simulink model "run_targeting"  (R2020a)
settings: Solver=ode23  StartTime=0.0  StopTime=7  MaxStep=0.01  RelTol=1e-6  EnableMultiTasking=on
InitFcn:
  | addpath('display/')
  | addpath('parameters/')
  | addpath('quadrotor_model')
  | addpath('tools/')
  | addpath('libs/RealTima_Pacer')
  | aerosonde_parameters
  | simulation_parameters
undefined symbols (not defined in the file or in its folder): drawQuadrotor, filter_freq, plotmavstatevariables, SAMPLE_TIME
libraries: simulink x23, realtime_pacer_lib x1
settings Model: Creator=beard  LastModifiedBy=andrey
settings DataIOCC: LimitDataPoints=on  SaveFormat=Array  SignalLoggingSaveFormat=ModelDataLogs  ReturnWorkspaceOutputs=off
settings OptimizationCC: ExpressionDepthLimit=2147483647  InitFltsAndDblsToZero=on  LifeSpan=inf
settings DebuggingCC: UnderspecifiedInitializationDetection=Classic  MergeDetectMultiDrivingBlocksExec=none  SolverPrmCheckMsg=warning  FcnCallInpInsideContextMsg=warning  AllowSymbolicDim=off  StateNameClashWarn=warning  SFUnexpectedBacktrackingDiag=warning  SFNoUnconditionalDefaultTransitionDiag=warning  SFExecutionAtInitializationDiag=none  ArithmeticOperatorsInVariantConditions=warning
settings HardwareCC: ProdBitPerPointer=32  ProdBitPerSizeT=32  ProdBitPerPtrDiffT=32  ProdLargestAtomicFloat=None  ProdIntDivRoundTo=Undefined  ProdEndianess=Unspecified  ProdWordSize=32  ProdHWDeviceType=32-bit Generic
settings ModelReferenceCC: PropagateSignalLabelsOutOfModel=off
settings SFSimCC: SimUseLocalCustomCode=off  CustomCodeUndefinedFunction=UseInterfaceOnly
settings RTWCC: RTWUseLocalCustomCode=off
settings CodeAppCC: StateflowObjectComments=on
settings GRTTargetCC: TargetLangStandard=C89/C90 (ANSI)  CombineOutputUpdateFcns=off  GRTInterface=on
settings ConfigComp: CovMetricSettings=dw  CovSaveCumulativeToWorkspaceVar=on  CovSaveSingleToWorkspaceVar=on  CovExternalEMLEnable=off  CovSFcnEnable=off

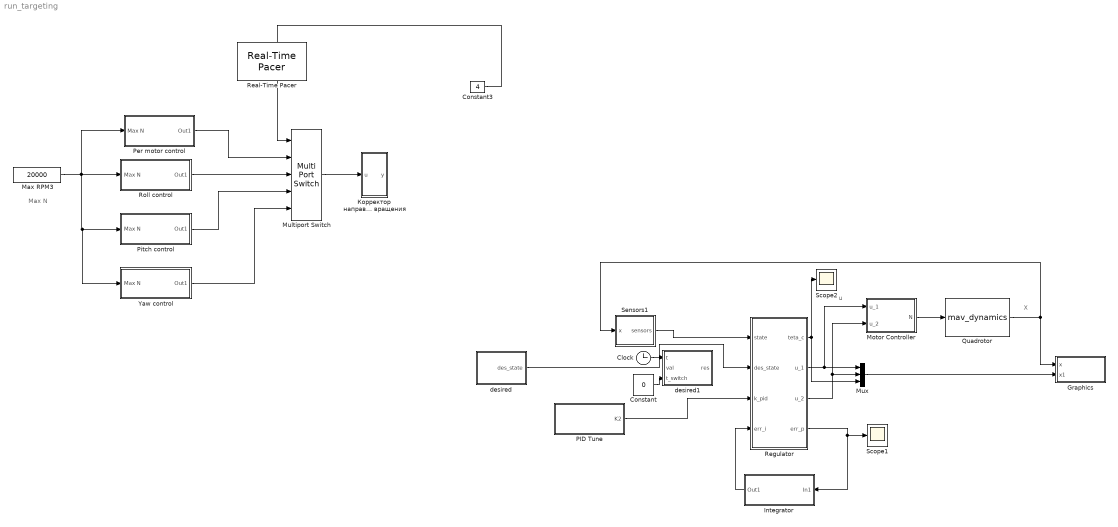
== system run_targeting ==
  note: X
  note: Max N
  note: u
  Clock : Clock
  Constant : Constant  Value=0
  Constant3 : Constant  Value=4
  Graphics : Subsystem
      mask Display: image(imread('../chap2/tv.jpg'))
  Integrator : Subsystem
  Max RPM3 : Constant  Value=20000  SampleTime=SAMPLE_TIME
  Motor Controller : MATLAB Function  TreatAsAtomicUnit=on
  Multiport Switch : MultiPortSwitch  Inputs=4
  Mux : Mux  Inputs=3
  PID Tune : Subsystem
  Per motor control : Subsystem
  Pitch control : Subsystem
  Quadrotor : S-Function  FunctionName=mav_dynamics  Parameters=MAV  SFunctionDeploymentMode=off  EnableBusSupport=off
  Real-Time Pacer : realtime_pacer_lib/Real-Time Pacer  simTimePerRealTime=1
  Regulator : MATLAB Function  TreatAsAtomicUnit=on
  Roll control : Subsystem
  Scope1 : Scope
  Scope2 : Scope
  Sensors1 : Subsystem
  Yaw control : Subsystem
  desired : MATLAB Function  TreatAsAtomicUnit=on
  desired1 : MATLAB Function  TreatAsAtomicUnit=on
  Корректор направлений вращения : MATLAB Function  TreatAsAtomicUnit=on
  wires:
  Quadrotor/1 -> Sensors1/1("x "), Graphics/1(x)
  Max RPM3/1 -> Roll control/1(Max N), Yaw control/1(Max N), Pitch control/1(Max N), Per motor control/1(Max N)
  Constant3/1 -> Multiport Switch/1
  Multiport Switch/1 -> Корректор направлений вращения/1(u)
  Per motor control/1(Out1) -> Multiport Switch/2
  Roll control/1(Out1) -> Multiport Switch/3
  Pitch control/1(Out1) -> Multiport Switch/4
  Yaw control/1(Out1) -> Multiport Switch/5
  Regulator/3(u_2) -> Motor Controller/2(u_2), Mux/2
  Regulator/2(u_1) -> Motor Controller/1(u_1), Mux/1
  Sensors1/1(sensors) -> Regulator/1(state)
  Motor Controller/1(N) -> Quadrotor/1
  Regulator/4(err_p) -> Integrator/1(In1), Scope1/1
  Regulator/1(teta_c) -> Mux/3, Scope2/1
  Integrator/1(Out1) -> Regulator/4(err_i)
  Mux/1 -> Graphics/2(x1)
  Clock/1 -> desired1/1(t)
  Constant/1 -> desired1/3(t_switch)
  PID Tune/1(K2) -> Regulator/3(k_pid)
  desired/1(des_state) -> Regulator/2(des_state)

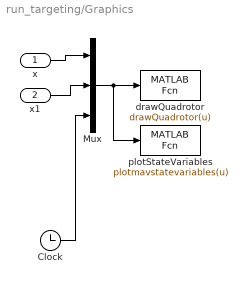
== system run_targeting/Graphics ==
  x : Inport
  x1 : Inport  Port=2
  Clock : Clock
  Mux : Mux  Inputs=3
  drawQuadrotor : MATLABFcn  MATLABFcn=drawQuadrotor(u)  OutputDimensions=0  SampleTime=0.1
  plotStateVariables : MATLABFcn  MATLABFcn=plotmavstatevariables(u)  OutputDimensions=0
  wires:
  x/1 -> Mux/1
  Mux/1 -> plotStateVariables/1, drawQuadrotor/1
  Clock/1 -> Mux/3
  x1/1 -> Mux/2

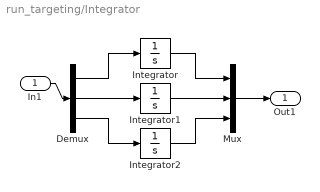
== system run_targeting/Integrator ==
  In1 : Inport
  Demux : Demux  Outputs=3
  Integrator : Integrator
  Integrator1 : Integrator
  Integrator2 : Integrator
  Mux : Mux  Inputs=3
  Out1 : Outport
  wires:
  In1/1 -> Demux/1
  Mux/1 -> Out1/1
  Integrator/1 -> Mux/1
  Integrator1/1 -> Mux/2
  Integrator2/1 -> Mux/3
  Demux/3 -> Integrator2/1
  Demux/2 -> Integrator1/1
  Demux/1 -> Integrator/1

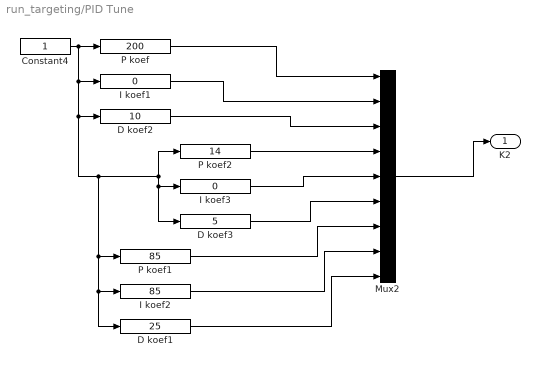
== system run_targeting/PID Tune ==
  Constant4 : Constant
  D koef1 : simulink/Math Operations/Slider Gain  gain=25  low=0  high=5000
  D koef2 : simulink/Math Operations/Slider Gain  gain=10  low=0  high=5000
  D koef3 : simulink/Math Operations/Slider Gain  gain=5  low=0  high=5000
  I koef1 : simulink/Math Operations/Slider Gain  gain=0  low=0  high=5000
  I koef2 : simulink/Math Operations/Slider Gain  gain=85  low=0  high=5000
  I koef3 : simulink/Math Operations/Slider Gain  gain=0  low=0  high=5000
  Mux2 : Mux  Inputs=9
  P koef : simulink/Math Operations/Slider Gain  gain=200  low=0  high=30000
  P koef1 : simulink/Math Operations/Slider Gain  gain=85  low=0  high=30000
  P koef2 : simulink/Math Operations/Slider Gain  gain=14  low=0  high=30000
  K2 : Outport
  wires:
  Mux2/1 -> K2/1
  Constant4/1 -> I koef1/1, I koef2/1, D koef1/1, P koef1/1, P koef2/1, I koef3/1, D koef3/1, D koef2/1, P koef/1
  P koef/1 -> Mux2/1
  I koef1/1 -> Mux2/2
  D koef2/1 -> Mux2/3
  P koef2/1 -> Mux2/4
  I koef3/1 -> Mux2/5
  D koef3/1 -> Mux2/6
  P koef1/1 -> Mux2/7
  I koef2/1 -> Mux2/8
  D koef1/1 -> Mux2/9

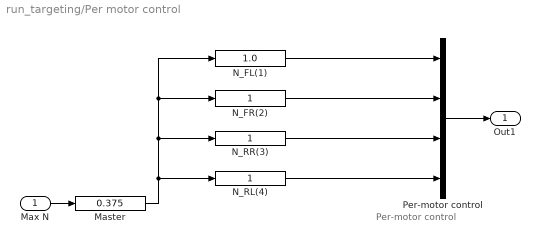
== system run_targeting/Per motor control ==
  note: Per-motor control
  Max N : Inport
  Master : simulink/Math Operations/Slider Gain  gain=0.375  low=0  high=1
  N_FL(1) : simulink/Math Operations/Slider Gain  gain=1.0  low=0  high=1
  N_FR(2) : simulink/Math Operations/Slider Gain  gain=1  low=0  high=1
  N_RL(4) : simulink/Math Operations/Slider Gain  gain=1  low=0  high=1
  N_RR(3) : simulink/Math Operations/Slider Gain  gain=1  low=0  high=1
  Per-motor control : Mux
  Out1 : Outport
  wires:
  N_RL(4)/1 -> Per-motor control/4
  N_FL(1)/1 -> Per-motor control/1
  N_FR(2)/1 -> Per-motor control/2
  Per-motor control/1 -> Out1/1
  Master/1 -> N_RL(4)/1, N_RR(3)/1, N_FR(2)/1, N_FL(1)/1
  N_RR(3)/1 -> Per-motor control/3
  Max N/1 -> Master/1

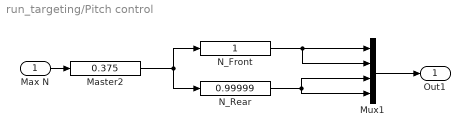
== system run_targeting/Pitch control ==
  Max N : Inport
  Master2 : simulink/Math Operations/Slider Gain  gain=0.375  low=0  high=1
  Mux1 : Mux
  N_Front : simulink/Math Operations/Slider Gain  gain=1  low=0  high=1
  N_Rear : simulink/Math Operations/Slider Gain  gain=0.99999  low=0  high=1
  Out1 : Outport
  wires:
  N_Rear/1 -> Mux1/3, Mux1/4
  Master2/1 -> N_Rear/1, N_Front/1
  N_Front/1 -> Mux1/2, Mux1/1
  Max N/1 -> Master2/1
  Mux1/1 -> Out1/1

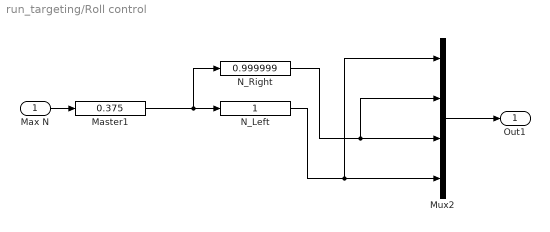
== system run_targeting/Roll control ==
  Max N : Inport
  Master1 : simulink/Math Operations/Slider Gain  gain=0.375  low=0  high=1
  Mux2 : Mux
  N_Left : simulink/Math Operations/Slider Gain  gain=1  low=0  high=1
  N_Right : simulink/Math Operations/Slider Gain  gain=0.999999  low=0  high=1
  Out1 : Outport
  wires:
  N_Right/1 -> Mux2/2, Mux2/3
  Master1/1 -> N_Left/1, N_Right/1
  N_Left/1 -> Mux2/1, Mux2/4
  Max N/1 -> Master1/1
  Mux2/1 -> Out1/1

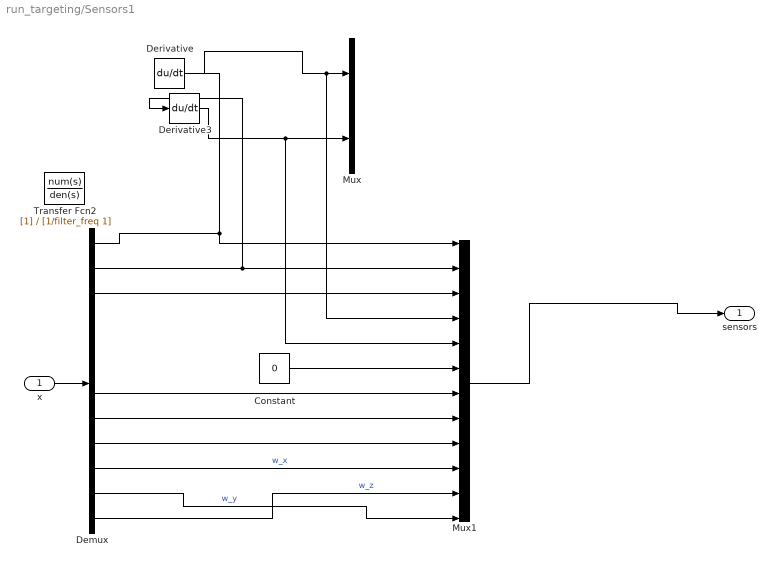
== system run_targeting/Sensors1 ==
  "x " : Inport
  Constant : Constant  Value=0
  Demux : Demux  Outputs=12
  Derivative : Derivative
  Derivative3 : Derivative
  Mux : Mux  Inputs=2
  Mux1 : Mux  Inputs=12
  Transfer Fcn2 : TransferFcn  Denominator=[1/filter_freq 1]
  sensors : Outport
  wires:
  "x "/1 -> Demux/1
  Demux/3 -> Mux1/3
  Constant/1 -> Mux1/6
  Demux/12 -> Mux1/11  "w_z"
  Demux/10 -> Mux1/10  "w_x"
  Demux/9 -> Mux1/9
  Demux/8 -> Mux1/8
  Demux/7 -> Mux1/7
  Demux/11 -> Mux1/12  "w_y"
  Mux1/1 -> sensors/1
  Derivative/1 -> Mux1/4, Mux/1
  Derivative3/1 -> Mux1/5, Mux/2
  Demux/1 -> Mux1/1, Derivative/1
  Demux/2 -> Mux1/2, Derivative3/1

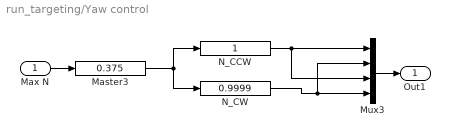
== system run_targeting/Yaw control ==
  Max N : Inport
  Master3 : simulink/Math Operations/Slider Gain  gain=0.375  low=0  high=1
  Mux3 : Mux
  N_CCW : simulink/Math Operations/Slider Gain  gain=1  low=0  high=1
  N_CW : simulink/Math Operations/Slider Gain  gain=0.9999  low=0  high=1
  Out1 : Outport
  wires:
  N_CCW/1 -> Mux3/3, Mux3/1
  Master3/1 -> N_CW/1, N_CCW/1
  N_CW/1 -> Mux3/2, Mux3/4
  Max N/1 -> Master3/1
  Mux3/1 -> Out1/1

== matlab function run_targeting/desired1 ==
  data: res output; t input; val input; t_switch input
function res = fcn(t, val, t_switch)
if t >= t_switch
    res = val;
else
    res = zeros(size(val));
end

== matlab function run_targeting/Корректор направлений вращения ==
  data: u input; y output
function y = fcn(u)

    y = [1 -1 1 -1]' .* u;

== matlab function run_targeting/Regulator ==
  data: teta_c output; state input; des_state input; k_pid input; u_1 output; u_2 output; err_p output; err_i input size=3; MAV parameter
function [teta_c, u_1, u_2, err_p] = fcn(state, des_state, k_pid, err_i, MAV)
    % прокси-функция для подключения функции-регулятора из .m файла.
    % позволяет держать код регулятора под контролем git
    % -----------------
    % MAV установлен как параметр: {Edit Data}->{Add}->{Type: Parameter}
    [teta_c, u_1, u_2, err_p] = regul(state, des_state, k_pid, err_i, MAV);

== matlab function run_targeting/Motor Controller ==
  data: N output; u_1 input; u_2 input
function N = fcn(u_1, u_2)

% teta_c = data(1);
% u_1 = data(2);
% u_2 = data(3);

NN = 0.25*[u_1+u_2 u_1+u_2 u_1-u_2 u_1-u_2]';
NN = max(NN, 0);
N = sqrt(NN);

== matlab function run_targeting/desired ==
  data: des_state output
function des_state = fcn()

pos = [0 1 0]';
vel = [0 0 0]';
acc = [0 0 0]';
des_state = [pos vel acc];
